simulink model "sim3"  (R2024a)
settings: Solver=FixedStepAuto  StartTime=0.0  StopTime=5.0  FixedStep=1e-3  RelTol=1e-3
InitFcn:
  | A=[0 1;
  |     -2 4];
  | b=[8;
  |     9];
  | Q=[3 0;
  |     0 4];
  | 
  | r1=1;
  | r2=4;
  | r3=10;
  | 
  | k1=0.5;
  | k2=1;
  | k3=2;
  | 
  | Q1=k1*Q;
  | Q2=k2*Q;
  | Q3=k3*Q;
  | 
  | % Q_1, r_i
  | K11=[-8.4524,10.0136];
  | K12=[-4.8045,5.8955];
  | K13=[-3.4856,4.4105];
  | 
  | % Q_2, r_i
  | K21=[-11.4926,13.4496];
  | K22=[-6.3100,7.5940];
  | K23=[-4.4233,5.4658];
  | 
  | % Q_3, r_i
  | K31=[-15.8004,18.3199];
  | K32=[-8.4524,10.0136];
  | K33=[-5.7660,6.9800];
libraries: matrix_library x9
settings Model: Creator=alexe  LastModifiedBy=alexe

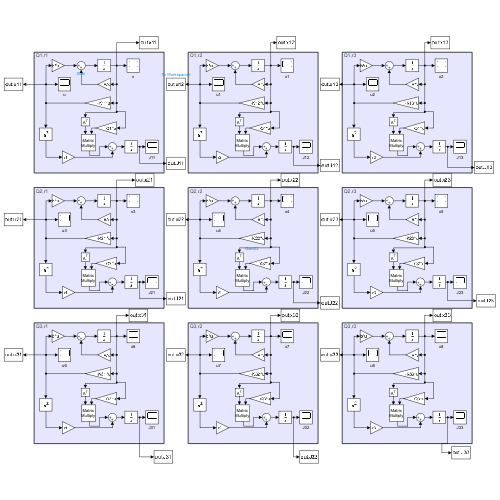
[thumbnail: Simulink's stored preview of the top-level diagram]
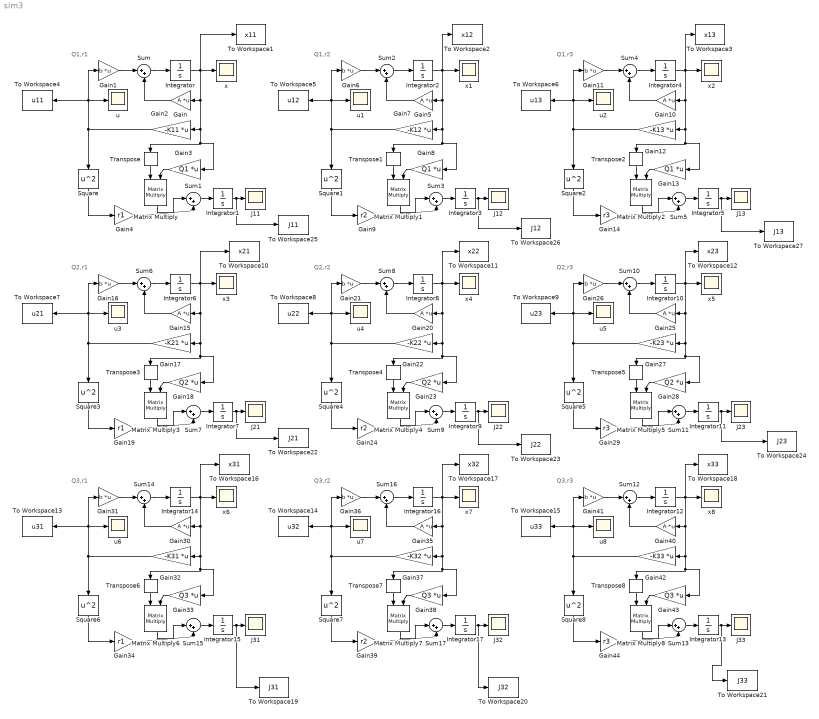
== system sim3 ==
  note: Q1,r1
  note: Q1,r2
  note: Q1,r3
  note: Q2,r1
  note: Q2,r2
  note: Q2,r3
  note: Q3,r2
  note: Q3,r1
  note: Q3,r3
  Gain{,5,10,15,20,25,30,35,40} (9 alike) : Gain  Gain=A  Multiplication=Matrix(K*u)
  Gain{1,6,11,16,21,26,31,36,41} (9 alike) : Gain  Gain=b  Multiplication=Matrix(K*u)
  Gain12 : Gain  Gain=-K13  Multiplication=Matrix(K*u)
  Gain13 : Gain  Gain=Q1  Multiplication=Matrix(K*u)
  Gain14 : Gain  Gain=r3
  Gain17 : Gain  Gain=-K21  Multiplication=Matrix(K*u)
  Gain18 : Gain  Gain=Q2  Multiplication=Matrix(K*u)
  Gain19 : Gain  Gain=r1
  Gain2 : Gain  Gain=-K11  Multiplication=Matrix(K*u)
  Gain22 : Gain  Gain=-K22  Multiplication=Matrix(K*u)
  Gain23 : Gain  Gain=Q2  Multiplication=Matrix(K*u)
  Gain24 : Gain  Gain=r2
  Gain27 : Gain  Gain=-K23  Multiplication=Matrix(K*u)
  Gain28 : Gain  Gain=Q2  Multiplication=Matrix(K*u)
  Gain29 : Gain  Gain=r3
  Gain3 : Gain  Gain=Q1  Multiplication=Matrix(K*u)
  Gain32 : Gain  Gain=-K31  Multiplication=Matrix(K*u)
  Gain33 : Gain  Gain=Q3  Multiplication=Matrix(K*u)
  Gain34 : Gain  Gain=r1
  Gain37 : Gain  Gain=-K32  Multiplication=Matrix(K*u)
  Gain38 : Gain  Gain=Q3  Multiplication=Matrix(K*u)
  Gain39 : Gain  Gain=r2
  Gain4 : Gain  Gain=r1
  Gain42 : Gain  Gain=-K33  Multiplication=Matrix(K*u)
  Gain43 : Gain  Gain=Q3  Multiplication=Matrix(K*u)
  Gain44 : Gain  Gain=r3
  Gain7 : Gain  Gain=-K12  Multiplication=Matrix(K*u)
  Gain8 : Gain  Gain=Q1  Multiplication=Matrix(K*u)
  Gain9 : Gain  Gain=r2
  Integrator{,2,4,6,8,10,12,14,16} (9 alike) : Integrator  InitialCondition=[1;0]
  Integrator{1,3,5,7,9,11,13,15,17} (9 alike) : Integrator
  J{11..13,21..23,31..33} (9 alike) : Scope
  Matrix Multiply{,1..8} (9 alike) : Product  Multiplication=Matrix(*)
  Square{,1..8} (9 alike) : Math  Operator=square
  Sum{,1..17} (18 alike) : Sum  Inputs=|++
  To Workspace1 : ToWorkspace  VariableName=x11  SaveFormat=Structure With Time  SampleTime=-1
  To Workspace10 : ToWorkspace  VariableName=x21  SaveFormat=Structure With Time  SampleTime=-1
  To Workspace11 : ToWorkspace  VariableName=x22  SaveFormat=Structure With Time  SampleTime=-1
  To Workspace12 : ToWorkspace  VariableName=x23  SaveFormat=Structure With Time  SampleTime=-1
  To Workspace13 : ToWorkspace  VariableName=u31  SaveFormat=Structure With Time  SampleTime=-1
  To Workspace14 : ToWorkspace  VariableName=u32  SaveFormat=Structure With Time  SampleTime=-1
  To Workspace15 : ToWorkspace  VariableName=u33  SaveFormat=Structure With Time  SampleTime=-1
  To Workspace16 : ToWorkspace  VariableName=x31  SaveFormat=Structure With Time  SampleTime=-1
  To Workspace17 : ToWorkspace  VariableName=x32  SaveFormat=Structure With Time  SampleTime=-1
  To Workspace18 : ToWorkspace  VariableName=x33  SaveFormat=Structure With Time  SampleTime=-1
  To Workspace19 : ToWorkspace  VariableName=J31  SaveFormat=Structure With Time  SampleTime=-1
  To Workspace2 : ToWorkspace  VariableName=x12  SaveFormat=Structure With Time  SampleTime=-1
  To Workspace20 : ToWorkspace  VariableName=J32  SaveFormat=Structure With Time  SampleTime=-1
  To Workspace21 : ToWorkspace  VariableName=J33  SaveFormat=Structure With Time  SampleTime=-1
  To Workspace22 : ToWorkspace  VariableName=J21  SaveFormat=Structure With Time  SampleTime=-1
  To Workspace23 : ToWorkspace  VariableName=J22  SaveFormat=Structure With Time  SampleTime=-1
  To Workspace24 : ToWorkspace  VariableName=J23  SaveFormat=Structure With Time  SampleTime=-1
  To Workspace25 : ToWorkspace  VariableName=J11  SaveFormat=Structure With Time  SampleTime=-1
  To Workspace26 : ToWorkspace  VariableName=J12  SaveFormat=Structure With Time  SampleTime=-1
  To Workspace27 : ToWorkspace  VariableName=J13  SaveFormat=Structure With Time  SampleTime=-1
  To Workspace3 : ToWorkspace  VariableName=x13  SaveFormat=Structure With Time  SampleTime=-1
  To Workspace4 : ToWorkspace  VariableName=u11  SaveFormat=Structure With Time  SampleTime=-1
  To Workspace5 : ToWorkspace  VariableName=u12  SaveFormat=Structure With Time  SampleTime=-1
  To Workspace6 : ToWorkspace  VariableName=u13  SaveFormat=Structure With Time  SampleTime=-1
  To Workspace7 : ToWorkspace  VariableName=u21  SaveFormat=Structure With Time  SampleTime=-1
  To Workspace8 : ToWorkspace  VariableName=u22  SaveFormat=Structure With Time  SampleTime=-1
  To Workspace9 : ToWorkspace  VariableName=u23  SaveFormat=Structure With Time  SampleTime=-1
  Transpose{,1..8} (9 alike) : matrix_library/Transpose
  u{,1..8} (9 alike) : Scope
  x{,1..8} (9 alike) : Scope
  wires:
  Integrator/1 -> To Workspace1/1, x/1, Transpose/1, Gain3/1, Gain2/1, Gain/1
  Gain/1 -> Sum/2
  Gain1/1 -> Sum/1
  Sum/1 -> Integrator/1
  Gain2/1 -> Square/1, To Workspace4/1, u/1, Gain1/1
  Matrix Multiply/1 -> Sum1/1
  Square/1 -> Gain4/1
  Gain4/1 -> Sum1/2
  Sum1/1 -> Integrator1/1
  Integrator1/1 -> To Workspace25/1, J11/1
  Transpose/1 -> Matrix Multiply/1
  Gain3/1 -> Matrix Multiply/2
  Transpose1/1 -> Matrix Multiply1/1
  Sum2/1 -> Integrator2/1
  Gain8/1 -> Matrix Multiply1/2
  Gain5/1 -> Sum2/2
  Gain9/1 -> Sum3/2
  Matrix Multiply1/1 -> Sum3/1
  Gain6/1 -> Sum2/1
  Gain7/1 -> Square1/1, To Workspace5/1, u1/1, Gain6/1
  Square1/1 -> Gain9/1
  Integrator2/1 -> x1/1, To Workspace2/1, Transpose1/1, Gain8/1, Gain7/1, Gain5/1
  Integrator3/1 -> To Workspace26/1, J12/1
  Sum3/1 -> Integrator3/1
  Transpose2/1 -> Matrix Multiply2/1
  Sum4/1 -> Integrator4/1
  Gain13/1 -> Matrix Multiply2/2
  Gain10/1 -> Sum4/2
  Gain14/1 -> Sum5/2
  Matrix Multiply2/1 -> Sum5/1
  Gain11/1 -> Sum4/1
  Gain12/1 -> Square2/1, To Workspace6/1, u2/1, Gain11/1
  Square2/1 -> Gain14/1
  Integrator4/1 -> To Workspace3/1, x2/1, Transpose2/1, Gain13/1, Gain12/1, Gain10/1
  Integrator5/1 -> To Workspace27/1, J13/1
  Sum5/1 -> Integrator5/1
  Transpose3/1 -> Matrix Multiply3/1
  Sum6/1 -> Integrator6/1
  Gain18/1 -> Matrix Multiply3/2
  Gain15/1 -> Sum6/2
  Gain19/1 -> Sum7/2
  Matrix Multiply3/1 -> Sum7/1
  Gain16/1 -> Sum6/1
  Gain17/1 -> Square3/1, To Workspace7/1, u3/1, Gain16/1
  Square3/1 -> Gain19/1
  Integrator6/1 -> To Workspace10/1, x3/1, Transpose3/1, Gain18/1, Gain17/1, Gain15/1
  Integrator7/1 -> To Workspace22/1, J21/1
  Sum7/1 -> Integrator7/1
  Integrator9/1 -> To Workspace23/1, J22/1
  Integrator8/1 -> To Workspace11/1, x4/1, Transpose4/1, Gain23/1, Gain22/1, Gain20/1
  Sum9/1 -> Integrator9/1
  Gain21/1 -> Sum8/1
  Gain24/1 -> Sum9/2
  Gain20/1 -> Sum8/2
  Gain23/1 -> Matrix Multiply4/2
  Sum8/1 -> Integrator8/1
  Transpose4/1 -> Matrix Multiply4/1
  Matrix Multiply4/1 -> Sum9/1
  Square4/1 -> Gain24/1
  Gain25/1 -> Sum10/2
  Gain28/1 -> Matrix Multiply5/2
  Sum10/1 -> Integrator10/1
  Transpose5/1 -> Matrix Multiply5/1
  Matrix Multiply5/1 -> Sum11/1
  Gain29/1 -> Sum11/2
  Integrator11/1 -> To Workspace24/1, J23/1
  Sum11/1 -> Integrator11/1
  Square5/1 -> Gain29/1
  Gain27/1 -> Square5/1, To Workspace9/1, u5/1, Gain26/1
  Integrator10/1 -> To Workspace12/1, x5/1, Transpose5/1, Gain28/1, Gain27/1, Gain25/1
  Gain26/1 -> Sum10/1
  Gain31/1 -> Sum14/1
  Matrix Multiply6/1 -> Sum15/1
  Gain34/1 -> Sum15/2
  Gain30/1 -> Sum14/2
  Gain33/1 -> Matrix Multiply6/2
  Sum14/1 -> Integrator14/1
  Transpose6/1 -> Matrix Multiply6/1
  Gain37/1 -> Square7/1, To Workspace14/1, u7/1, Gain36/1
  Matrix Multiply7/1 -> Sum17/1
  Gain38/1 -> Matrix Multiply7/2
  Gain35/1 -> Sum16/2
  Sum17/1 -> Integrator17/1
  Sum15/1 -> Integrator15/1
  Square6/1 -> Gain34/1
  Gain39/1 -> Sum17/2
  Gain32/1 -> Square6/1, To Workspace13/1, u6/1, Gain31/1
  Integrator17/1 -> To Workspace20/1, J32/1
  Integrator12/1 -> To Workspace18/1, x8/1, Transpose8/1, Gain43/1, Gain42/1, Gain40/1
  Gain41/1 -> Sum12/1
  Sum13/1 -> Integrator13/1
  Sum16/1 -> Integrator16/1
  Transpose8/1 -> Matrix Multiply8/1
  Integrator13/1 -> To Workspace21/1, J33/1
  Integrator16/1 -> To Workspace17/1, x7/1, Transpose7/1, Gain38/1, Gain37/1, Gain35/1
  Gain43/1 -> Matrix Multiply8/2
  Gain36/1 -> Sum16/1
  Transpose7/1 -> Matrix Multiply7/1
  Matrix Multiply8/1 -> Sum13/1
  Gain42/1 -> Square8/1, To Workspace15/1, u8/1, Gain41/1
  Square8/1 -> Gain44/1
  Square7/1 -> Gain39/1
  Gain40/1 -> Sum12/2
  Integrator15/1 -> To Workspace19/1, J31/1
  Sum12/1 -> Integrator12/1
  Integrator14/1 -> To Workspace16/1, x6/1, Transpose6/1, Gain33/1, Gain32/1, Gain30/1
  Gain44/1 -> Sum13/2
  Gain22/1 -> Square4/1, To Workspace8/1, u4/1, Gain21/1
